simulink model "Prvi2012B"  (R2012b)
settings: Solver=ode45  SolverMode=SingleTasking  StartTime=0.0  StopTime=500  RelTol=1e-3
settings Model: CovMetricSettings=dwe  CovHtmlReporting=off  covSaveCumulativeToWorkspaceVar=off  CovSaveSingleToWorkspaceVar=off  CovExternalEMLEnable=on  Creator=Aldin  LastModifiedBy=Aldin
settings DataIOCC: LimitDataPoints=off  SaveFormat=StructureWithTime  ReturnWorkspaceOutputs=on
settings OptimizationCC: ExpressionDepthLimit=128
settings DebuggingCC: UnderspecifiedInitializationDetection=Simplified  MergeDetectMultiDrivingBlocksExec=error  SolverPrmCheckMsg=none  FrameProcessingCompatibilityMsg=error  StateNameClashWarn=none  SFUnexpectedBacktrackingDiag=error  SFNoUnconditionalDefaultTransitionDiag=error
settings HardwareCC: ProdBitPerPointer=64  ProdLargestAtomicFloat=Float  ProdIntDivRoundTo=Zero  ProdEndianess=LittleEndian  ProdHWDeviceType=Specified
settings ModelReferenceCC: PropagateSignalLabelsOutOfModel=on
settings SFSimCC: SimUseLocalCustomCode=on
settings RTWCC: RTWUseLocalCustomCode=on
settings CodeAppCC: CustomSymbolStrType=$N$R$M_T
settings GRTTargetCC: CodeReplacementLibrary=C99 (ISO)

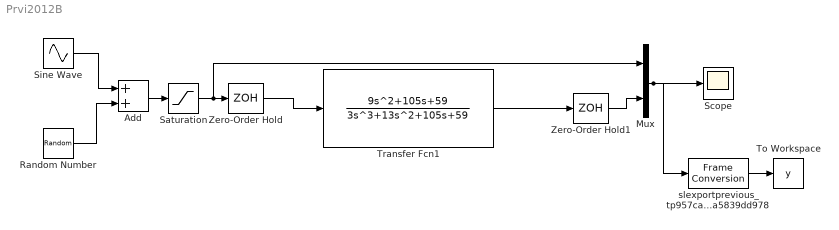
== system Prvi2012B ==
  Add : Sum
  Mux : Mux  Inputs=2
  Random Number : RandomNumber  Variance=0.1  SampleTime=0.1
  Saturation : Saturate  UpperLimit=5  LowerLimit=-5
  Scope : Scope
      settings: TimeRange=auto  MaxDataPoints=5000  SaveToWorkspace=off  SaveName=ScopeData  YMin=-6.132  YMax=6.03775  SampleTime=-1
  Sine Wave : Sin  Amplitude=4  Frequency=0.025  SampleTime=0.1
  To Workspace : ToWorkspace  VariableName=y  SampleTime=-1
  Transfer Fcn1 : TransferFcn  Numerator=[9 105 59]  Denominator=[3 13 105 59]
  Zero-Order Hold : ZeroOrderHold  SampleTime=0.1
  Zero-Order Hold1 : ZeroOrderHold  SampleTime=0.1
  slexportprevious_tp957ca115_3d01_497d_81a1_30a5839dd978 : FrameConversion  OutFrame=Sample-based
  wires:
  Saturation/1 -> Mux/1, Zero-Order Hold/1
  Random Number/1 -> Add/2
  Mux/1 -> Scope/1, slexportprevious_tp957ca115_3d01_497d_81a1_30a5839dd978/1
  Zero-Order Hold/1 -> Transfer Fcn1/1
  Zero-Order Hold1/1 -> Mux/2
  Sine Wave/1 -> Add/1
  Transfer Fcn1/1 -> Zero-Order Hold1/1
  Add/1 -> Saturation/1
  slexportprevious_tp957ca115_3d01_497d_81a1_30a5839dd978/1 -> To Workspace/1
